simulink model "controller_3dof"  (R2023a)
settings: Solver=FixedStepAuto  StartTime=0.0  StopTime=inf  FixedStep=0.01  RelTol=1e-3  EnableMultiTasking=on
undefined symbols (not defined in the file): dev, DiscIntNeverNeededParam, IMU_w_b_bias, Kv, Kx, Main, meas_pole, P0_phth, P0_ps, pwm_output0, Q_phth, q_ps, R_phth, r_ps, Rz, Ts_EKF_integr, Ts_EKF_meas, Ts_slk, x0_phth, x0_ps
libraries: px4Sensorslib x4, px4lib x1, px4uORBlib x1, sharedtransform x1
settings Model: SimulationMode=external  ExtModeTrigDuration=10  Creator=ArriGE66  LastModifiedBy=User
settings SolverCC: PositivePriorityOrder=on
settings OptimizationCC: EnhancedBackFolding=on  PassReuseOutputArgsAs=Individual arguments  ZeroExternalMemoryAtStartup=off  ZeroInternalMemoryAtStartup=off  MaxStackSize=64  OptimizeBlockOrder=speed  DifferentSizesBufferReuse=on  OptimizationCustomize=off  EfficientTunableParamExpr=on
settings DebuggingCC: ParameterTunabilityLossMsg=error
settings HardwareCC: ProdBitPerPointer=32  ProdBitPerSizeT=32  ProdBitPerPtrDiffT=32  ProdLargestAtomicInteger=Long  ProdLargestAtomicFloat=Double  ProdWordSize=32  ProdLongLongMode=on  ProdHWDeviceType=ARM Compatible->ARM Cortex
settings SFSimCC: MATLABDynamicMemAlloc=off  SimTargetLang=C++
settings RTWCC: Description=Embedded Coder  SystemTargetFile=ert.tlc  HardwareBoard=PX4 Cube Orange  TemplateMakefile=ert_default_tmf  Toolchain=GNU Tools for PX4 Autopilots  TargetLang=C++
settings CodeAppCC: ForceParamTrailComments=on  IgnoreCustomStorageClasses=off  OperatorAnnotations=on  SimulinkDataObjDesc=on  SFDataObjDesc=on  InsertBlockDesc=on
settings ERTTargetCC: ExtMode=on  ExtModeTransport=3  ExtModeStaticAlloc=on  ExtModeStaticAllocSize=1024  ExtModeMexFile=ext_xcp  ExtModeMexArgs=1 COM10 3000000  ExtModeIntrfLevel=Level2 - Open

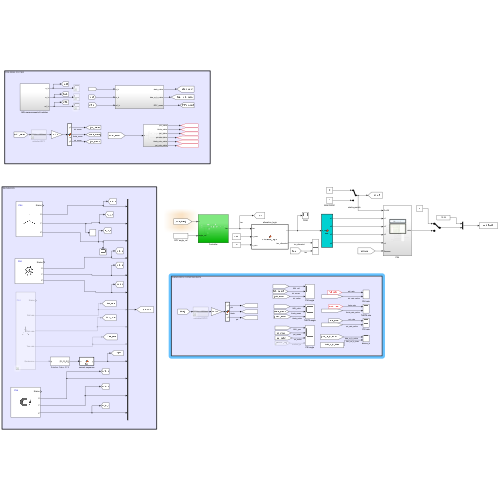
[thumbnail: Simulink's stored preview of the top-level diagram]
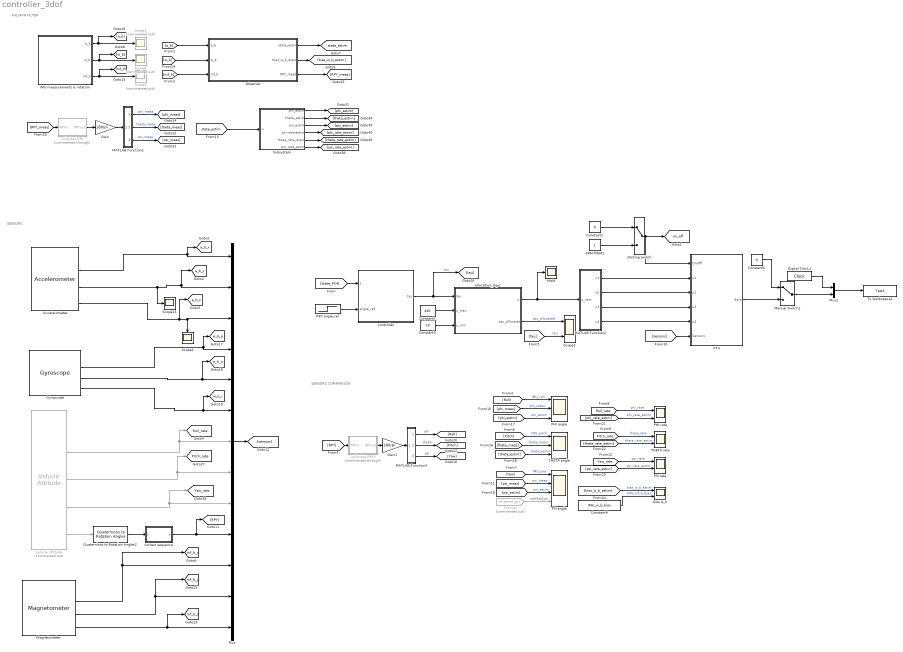
== system controller_3dof ==
  note: KALMAN FILTER
  note: SENSORS COMPARISON
  note: SENSORS
  ARM PWM1 : Constant  OutDataTypeStr=boolean  SampleTime=0.01
  Accelerometer : px4Sensorslib/Accelerometer  uorbTimeStamp=off  BlockingMode=off  BlockTimeout=1e-3  sampleTime=1/100
  Constant1 : Constant  Value=450  SampleTime=0.01
  Constant2 : Constant  Value=0  OutDataTypeStr=boolean
  Constant3 : Constant  Value=10  SampleTime=0.01
  Constant4 : Constant  Value=IMU_w_b_bias
  Constant6 : Constant  Value=0  OutDataTypeStr=boolean
  Controller : Subsystem
  Digital Clock1 : DigitalClock  SampleTime=0.01
  From20 : From  Commented=on  GotoTag=method_ps
  Gain : Gain  Gain=180/pi
  Gain1 : Gain  Gain=180/pi
  Gyroscope : px4Sensorslib/Gyroscope  uorbTimeStamp=off  BlockingMode=off  BlockTimeout=1e-3  sampleTime=1/100
  IMU measurements & rotation : Subsystem
  MATLAB Function1 : MATLAB Function  TreatAsAtomicUnit=on
  MATLAB Function2 : MATLAB Function  TreatAsAtomicUnit=on
  MATLAB Function3 : MATLAB Function  TreatAsAtomicUnit=on
  Magnetometer : px4Sensorslib/Magnetometer  uorbTimeStamp=off  BlockingMode=off  BlockTimeout=1e-3  sampleTime=0.01
  Manual Switch2 : ManualSwitch
  Mux : Mux  Inputs=13
  Mux2 : Mux  Inputs=2
  Observer : Subsystem
  PHI angle : Scope  NumInputPorts=3
  PHI rate : Scope  NumInputPorts=2
  PSI angle : Scope  NumInputPorts=4
  PSI rate : Scope  NumInputPorts=2
  PWM : Scope
  PX4 : Subsystem
  Quaternions to Rotation Angles2 : sharedtransform/Quaternions to Rotation Angles  rotationOrder=ZYX  aMode=aMode
  RPY angle_ref : Step  Time=0  After=zeros(3,1)  SampleTime=0.01
  Scope1 : Scope
  Scope13 : Scope
  Scope2 : Scope  NumInputPorts=2
  Scope3 : Scope  Commented=on
  Scope8 : Scope  Commented=on
  Scope9 : Scope  Commented=on
  Subsystem : Subsystem
  THETA angle : Scope  NumInputPorts=3
  THETA rate : Scope  NumInputPorts=2
  To Workspace1 : ToWorkspace  VariableName=Test1  SampleTime=-1
      settings: Save2DSignal=2-D array (concatenate along first dimension)
  Vehicle Attitude : px4Sensorslib/Vehicle Attitude  Commented=on  rollRate=on  pitchRate=on  yawRate=on  quaternion=on  uorbTimeStamp=off  BlockingMode=off  BlockTimeout=0.001  sampleTime=1/100
  allocation_logic : MATLAB Function  TreatAsAtomicUnit=on
  bias w_b : Scope  NumInputPorts=2
  correct sequence : MATLAB Function  TreatAsAtomicUnit=on
  starting switch : ManualSwitch
  unlimited RPY : Subsystem  Commented=through
  unlimited RPY2 : Subsystem  Commented=through
  tag scope: Pitch_rate=global, Roll_rate=global, Yaw_rate=global, a_b_x=global, a_b_y=global, a_b_z=global, mf_b_x=global, mf_b_y=global, mf_b_z=global, on_off=global, state_estim=global, w_b_p=global, w_b_q=global, w_b_r=global
  wires:
  MATLAB Function2/4(u4) -> PX4/5(u4)
  MATLAB Function2/3(u3) -> PX4/4(u3)
  MATLAB Function2/2(u2) -> PX4/3(u2)
  MATLAB Function2/1(u1) -> PX4/2(u1)
  allocation_logic/2(tau_allocated) -> Scope2/1  "tau_allocated"
  allocation_logic/1(u) -> PWM/1, MATLAB Function2/1(u_vect)
  Controller/1(tau) -> [tau], allocation_logic/1(tau)  "tau"
  RPY angle_ref/1 -> Controller/2(angle_ref)
  [tau] -> Scope2/2  "tau"
  [state_PX4] -> Controller/1(x)
  Constant3/1 -> allocation_logic/3(u_min)
  Subsystem/5(theta_rate_estim) -> [theta_rate_estim]
  Subsystem/6(psi_rate_estim) -> [psi_rate_estim]
  Subsystem/1(phi_estim) -> [phi_estim]
  Subsystem/3(psi_estim) -> [psi_estim]
  [state_estim] -> Subsystem/1(u)
  unlimited RPY2/1(RPYout) -> Gain1/1
  Observer/3(RPY_meas) -> [RPY_meas]
  IMU measurements & rotation/2(w_b) -> [w_b], Scope8/1
  MATLAB Function3/3(y3) -> [Yaw]  "psi"
  [theta_estim] -> THETA angle/3  "theta_estim"
  From20/1 -> PSI angle/4  "method_ps"
  [phi_rate_estim] -> PHI rate/2  "phi_rate_estim"
  Observer/1(state_estim) -> [state_estim]
  Mux/1 -> [sensors]
  starting switch/1 -> PX4/1(On/Off), [on_off]
  [Yaw] -> PSI angle/1  "IMU_yaw"
  Gyroscope/2 -> [w_b_p], Mux/4
  IMU measurements & rotation/3(mf_b) -> [mf_b], Scope9/1
  IMU measurements & rotation/1(a_b) -> [a_b], Scope3/1
  [w_b] -> Observer/2(w_b)
  [mf_b] -> Observer/3(mf_b)
  [a_b] -> Observer/1(a_b)
  [psi_rate_estim] -> PSI rate/2  "psi_rate_estim"
  unlimited RPY/1(RPYout) -> Gain/1
  Gyroscope/3 -> [w_b_q], Mux/5
  [Roll] -> PHI angle/1  "IMU_roll"
  [psi_estim] -> PSI angle/3  "psi_estim"
  [psi_meas] -> PSI angle/2  "psi_meas"
  Observer/2(bias_w_b_estim) -> [bias_w_b_estim]
  Constant4/1 -> bias w_b/2  "IMU_mf_b_bias"
  Manual Switch2/1 -> Mux2/2
  [phi_estim] -> PHI angle/3  "phi_estim"
  correct sequence/1(y) -> [RPY], Mux/10
  [RPY] -> unlimited RPY2/1(RPYin)
  Vehicle Attitude/5 -> Quaternions to Rotation Angles2/1
  [Pitch] -> THETA angle/1  "IMU_pitch"
  MATLAB Function3/2(y2) -> [Pitch]  "theta"
  Magnetometer/3 -> Mux/12, [mf_b_y]
  Gain1/1 -> MATLAB Function3/1(u)
  [Pitch_rate] -> THETA rate/1  "theta_rate"
  [bias_w_b_estim] -> bias w_b/1  "bias_w_b_estim"
  MATLAB Function1/1(y1) -> [phi_meas]  "phi_meas"
  [theta_rate_estim] -> THETA rate/2  "theta_rate_estim"
  [phi_meas] -> PHI angle/2  "phi_meas"
  Vehicle Attitude/2 -> [Roll_rate], Mux/7
  PX4/1(data) -> Manual Switch2/2
  Gain/1 -> MATLAB Function1/1(u)
  [RPY_meas] -> unlimited RPY/1(RPYin)
  Quaternions to Rotation Angles2/1 -> correct sequence/1(u)
  Subsystem/4(phi-rate-estim) -> [phi_rate_estim]
  Digital Clock1/1 -> Mux2/1
  Constant2/1 -> starting switch/1
  Vehicle Attitude/3 -> [Pitch_rate], Mux/8
  Constant6/1 -> Manual Switch2/1
  MATLAB Function1/3(y3) -> [psi_meas]  "psi_meas"
  [theta_meas] -> THETA angle/2  "theta_meas"
  Mux2/1 -> To Workspace1/1
  MATLAB Function1/2(y2) -> [theta_meas]  "theta_meas"
  [sensors] -> PX4/6(Sensors)
  Magnetometer/2 -> [mf_b_x], Mux/11
  Magnetometer/4 -> [mf_b_z], Mux/13
  [Yaw_rate] -> PSI rate/1  "psi_rate"
  Subsystem/2(theta_estim) -> [theta_estim]
  Vehicle Attitude/4 -> [Yaw_rate], Mux/9
  Gyroscope/4 -> [w_b_r], Mux/6
  Accelerometer/3 -> Scope13/1, [a_b_y], Mux/2
  MATLAB Function3/1(y1) -> [Roll]  "phi"
  ARM PWM1/1 -> starting switch/2
  [Roll_rate] -> PHI rate/1  "phi_rate"
  Accelerometer/2 -> [a_b_x], Mux/1
  Accelerometer/4 -> [a_b_z], Mux/3, Scope1/1
  Constant1/1 -> allocation_logic/2(u_max)

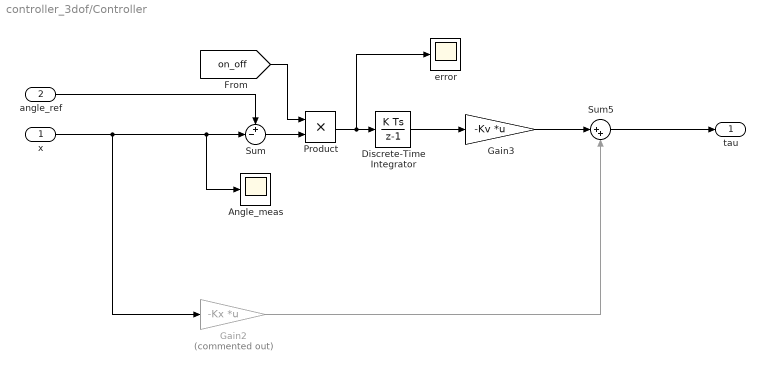
== system controller_3dof/Controller ==
  x : Inport
  angle_ref : Inport  Port=2
  Angle_meas : Scope
  Discrete-Time Integrator : DiscreteIntegrator  SampleTime=Ts_slk  ICPrevOutput=DiscIntNeverNeededParam  ICPrevScaledInput=DiscIntNeverNeededParam
  Gain2 : Gain  Commented=on  Gain=-Kx  Multiplication=Matrix(K*u)
  Gain3 : Gain  Gain=-Kv  Multiplication=Matrix(K*u)
  Product : Product
  Sum : Sum  Inputs=+-|
  Sum5 : Sum  Inputs=|++
  error : Scope
  tau : Outport
  wires:
  x/1 -> Angle_meas/1, Sum/2, Gain2/1
  Sum5/1 -> tau/1
  angle_ref/1 -> Sum/1
  Discrete-Time Integrator/1 -> Gain3/1
  Gain3/1 -> Sum5/1
  Gain2/1 -> Sum5/2
  Sum/1 -> Product/2
  [on_off] -> Product/1
  Product/1 -> error/1, Discrete-Time Integrator/1

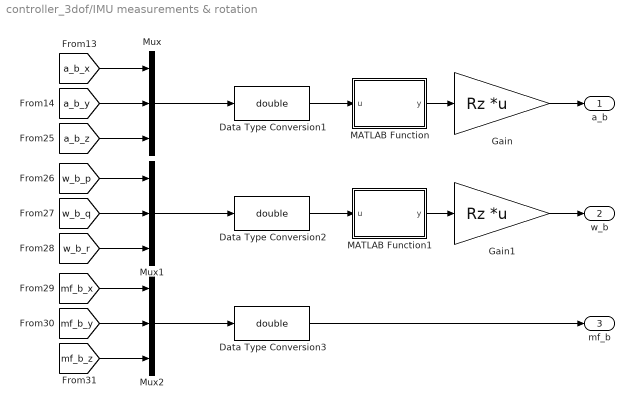
== system controller_3dof/IMU measurements & rotation ==
  Data Type Conversion1 : DataTypeConversion  OutDataTypeStr=double  SaturateOnIntegerOverflow=off  RndMeth=Floor
  Data Type Conversion2 : DataTypeConversion  OutDataTypeStr=double  SaturateOnIntegerOverflow=off  RndMeth=Floor
  Data Type Conversion3 : DataTypeConversion  OutDataTypeStr=double  SaturateOnIntegerOverflow=off  RndMeth=Floor
  Gain : Gain  Gain=Rz  Multiplication=Matrix(K*u) (u vector)
  Gain1 : Gain  Gain=Rz  Multiplication=Matrix(K*u) (u vector)
  MATLAB Function : MATLAB Function  TreatAsAtomicUnit=on
  MATLAB Function1 : MATLAB Function  TreatAsAtomicUnit=on
  Mux : Mux  Inputs=3
  Mux1 : Mux  Inputs=3
  Mux2 : Mux  Inputs=3
  a_b : Outport
  w_b : Outport  Port=2
  mf_b : Outport  Port=3
  wires:
  Mux2/1 -> Data Type Conversion3/1
  Gain/1 -> a_b/1
  Mux1/1 -> Data Type Conversion2/1
  MATLAB Function/1(y) -> Gain/1
  Mux/1 -> Data Type Conversion1/1
  MATLAB Function1/1(y) -> Gain1/1
  Gain1/1 -> w_b/1
  [a_b_x] -> Mux/1
  [a_b_y] -> Mux/2
  [a_b_z] -> Mux/3
  [w_b_p] -> Mux1/1
  [w_b_q] -> Mux1/2
  [w_b_r] -> Mux1/3
  [mf_b_x] -> Mux2/1
  [mf_b_y] -> Mux2/2
  [mf_b_z] -> Mux2/3
  Data Type Conversion1/1 -> MATLAB Function/1(u)
  Data Type Conversion2/1 -> MATLAB Function1/1(u)
  Data Type Conversion3/1 -> mf_b/1

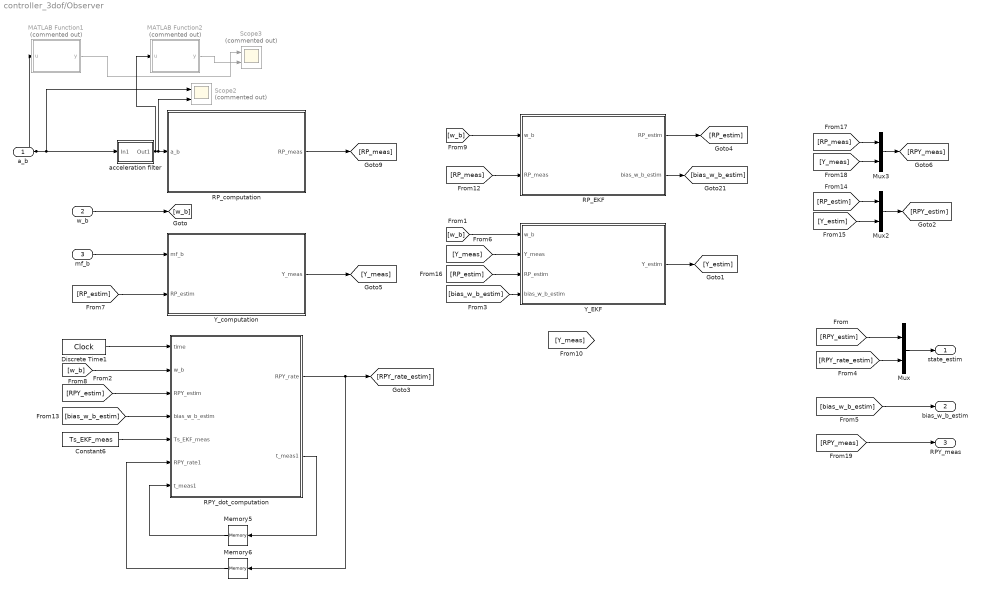
== system controller_3dof/Observer ==
  a_b : Inport
  w_b : Inport  Port=2
  mf_b : Inport  Port=3
  Constant6 : Constant  Value=Ts_EKF_meas
  Discrete Time1 : DigitalClock  SampleTime=Ts_slk
  MATLAB Function1 : MATLAB Function  Commented=on  TreatAsAtomicUnit=on
  MATLAB Function2 : MATLAB Function  Commented=on  TreatAsAtomicUnit=on
  Memory5 : Memory
  Memory6 : Memory
  Mux : Mux  Inputs=2
  Mux2 : Mux  Inputs=2
  Mux3 : Mux  Inputs=2
  RPY_dot_computation : MATLAB Function  TreatAsAtomicUnit=on
  RP_EKF : Subsystem
  RP_computation : MATLAB Function  TreatAsAtomicUnit=on
  Scope2 : Scope  Commented=on  NumInputPorts=2
  Scope3 : Scope  Commented=on  NumInputPorts=2
  Y_EKF : Subsystem
  Y_computation : MATLAB Function  TreatAsAtomicUnit=on
  acceleration filter : Subsystem  mask{p=meas_pole}
      mask prompts: p "pole (p)"
  state_estim : Outport
  bias_w_b_estim : Outport  Port=2
  RPY_meas : Outport  Port=3
  wires:
  Memory5/1 -> RPY_dot_computation/7("t_meas1 ")
  Discrete Time1/1 -> RPY_dot_computation/1(time)
  RPY_dot_computation/2(t_meas1) -> Memory5/1
  [w_b] -> RPY_dot_computation/2(w_b)
  Memory6/1 -> RPY_dot_computation/6(RPY_rate1)
  RPY_dot_computation/1(RPY_rate) -> Memory6/1, [RPY_rate_estim]
  Constant6/1 -> RPY_dot_computation/5(Ts_EKF_meas)
  [RPY_estim] -> RPY_dot_computation/3(RPY_estim)
  [bias_w_b_estim] -> RPY_dot_computation/4(bias_w_b_estim)
  [RPY_estim] -> Mux/1
  [RPY_rate_estim] -> Mux/2
  Mux/1 -> state_estim/1
  [bias_w_b_estim] -> bias_w_b_estim/1
  [RPY_meas] -> RPY_meas/1
  RP_EKF/2(bias_w_b_estim) -> [bias_w_b_estim]
  [RP_estim] -> Y_computation/2(RP_estim)
  [Y_meas] -> Y_EKF/2(Y_meas)
  Y_computation/1(Y_meas) -> [Y_meas]
  RP_EKF/1(RP_estim) -> [RP_estim]
  [w_b] -> Y_EKF/1(w_b)
  RP_computation/1(RP_meas) -> [RP_meas]
  [RP_meas] -> RP_EKF/2(RP_meas)
  [w_b] -> RP_EKF/1(w_b)
  Y_EKF/1(Y_estim) -> [Y_estim]
  mf_b/1 -> Y_computation/1(mf_b)
  w_b/1 -> [w_b]
  [bias_w_b_estim] -> Y_EKF/4(bias_w_b_estim)
  [RP_estim] -> Mux2/1
  [Y_estim] -> Mux2/2
  Mux2/1 -> [RPY_estim]
  [RP_estim] -> Y_EKF/3(RP_estim)
  [RP_meas] -> Mux3/1
  Mux3/1 -> [RPY_meas]
  [Y_meas] -> Mux3/2
  MATLAB Function1/1(y) -> Scope3/1
  a_b/1 -> Scope2/1, acceleration filter/1(In1), MATLAB Function1/1(u)
  MATLAB Function2/1(y) -> Scope3/2
  acceleration filter/1(Out1) -> MATLAB Function2/1(u), Scope2/2, RP_computation/1(a_b)

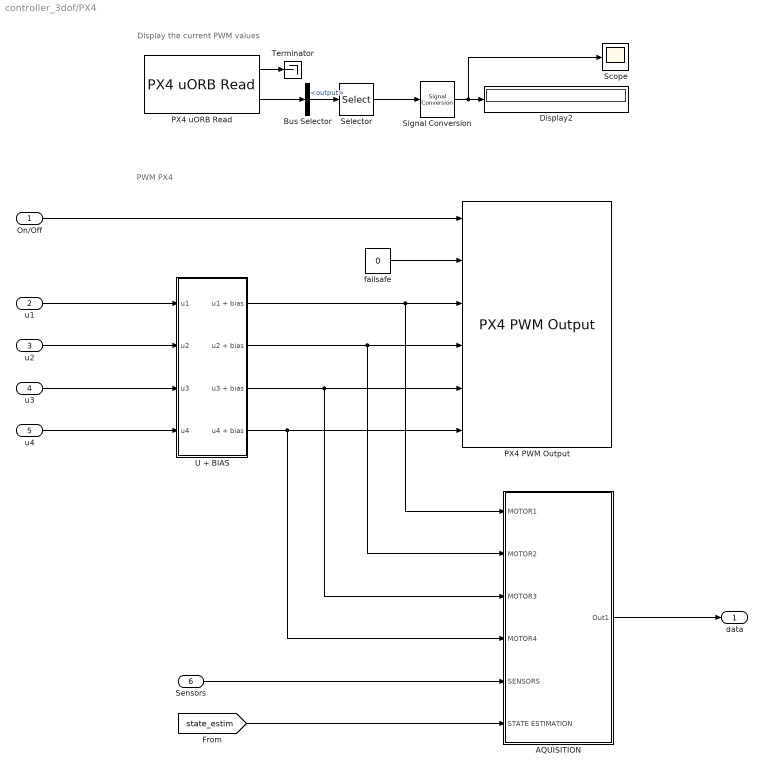
== system controller_3dof/PX4 ==
  note: PWM PX4
  note: Display the current PWM values
  On/Off : Inport
  u1 : Inport  Port=2
  u2 : Inport  Port=3
  u3 : Inport  Port=4
  u4 : Inport  Port=5
  Sensors : Inport  Port=6
  AQUISITION : Subsystem
  Bus Selector : BusSelector  OutputSignals=output
  Display2 : Display
  PX4 PWM Output : px4lib/PX4 PWM Output  pwmDevice=Main (/dev/pwm_output0)  pwmChannel1_=on  pwmChannel2_=on  pwmChannel3_=on  pwmChannel4_=on  pwmChannel5_=off  pwmChannel6_=off  pwmChannel7_=off  pwmChannel8_=off  forceTerminateFailsafe=off  outputErrorStatus=on
  PX4 uORB Read : px4uORBlib/PX4 uORB Read  uORBTopic=actuator_outputs  selectInstance=actuator_outputs  SampleTime=0.01  BlockingMode=off  BlockTimeout=1e-3
  Scope : Scope
  Selector : Selector  InputPortWidth=16  IndexOptions=Index vector (dialog)  Indices=[1 2]  OutputSizes=1
  Signal Conversion : SignalConversion  OverrideOpt=off
  Terminator : Terminator
  U + BIAS : Subsystem
  failsafe : Constant  Value=0  OutDataTypeStr=boolean  SampleTime=0.01
  data : Outport
  wires:
  failsafe/1 -> PX4 PWM Output/2
  U + BIAS/2(u2 + bias) -> AQUISITION/2(MOTOR2), PX4 PWM Output/4
  U + BIAS/4(u4 + bias) -> AQUISITION/4(MOTOR4), PX4 PWM Output/6
  U + BIAS/3(u3 + bias) -> AQUISITION/3(MOTOR3), PX4 PWM Output/5
  U + BIAS/1(u1 + bias) -> AQUISITION/1(MOTOR1), PX4 PWM Output/3
  Sensors/1 -> AQUISITION/5(SENSORS)
  On/Off/1 -> PX4 PWM Output/1
  u4/1 -> U + BIAS/4(u4)
  AQUISITION/1(Out1) -> data/1
  u1/1 -> U + BIAS/1(u1)
  u2/1 -> U + BIAS/2(u2)
  u3/1 -> U + BIAS/3(u3)
  [state_estim] -> AQUISITION/6(STATE ESTIMATION)
  Selector/1 -> Signal Conversion/1
  PX4 uORB Read/2 -> Bus Selector/1
  Signal Conversion/1 -> Scope/1, Display2/1
  Bus Selector/1 -> Selector/1  "<output>"
  PX4 uORB Read/1 -> Terminator/1

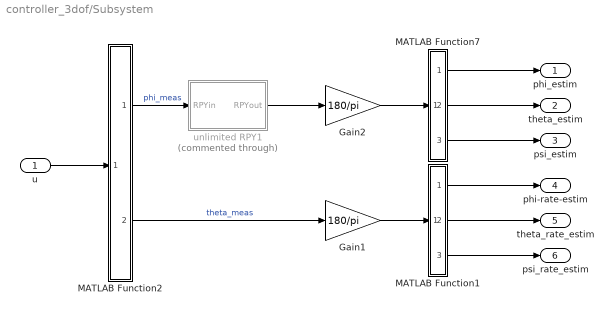
== system controller_3dof/Subsystem ==
  u : Inport
  Gain1 : Gain  Gain=180/pi
  Gain2 : Gain  Gain=180/pi
  MATLAB Function1 : MATLAB Function  TreatAsAtomicUnit=on
  MATLAB Function2 : MATLAB Function  TreatAsAtomicUnit=on
  MATLAB Function7 : MATLAB Function  TreatAsAtomicUnit=on
  unlimited RPY1 : Subsystem  Commented=through
  phi_estim : Outport
  theta_estim : Outport  Port=2
  psi_estim : Outport  Port=3
  phi-rate-estim : Outport  Port=4
  theta_rate_estim : Outport  Port=5
  psi_rate_estim : Outport  Port=6
  wires:
  u/1 -> MATLAB Function2/1(u)
  MATLAB Function2/2(y2) -> Gain1/1  "theta_meas"
  MATLAB Function2/1(y1) -> unlimited RPY1/1(RPYin)  "phi_meas"
  MATLAB Function7/2(y2) -> theta_estim/1
  MATLAB Function7/1(y1) -> phi_estim/1
  MATLAB Function7/3(y3) -> psi_estim/1
  unlimited RPY1/1(RPYout) -> Gain2/1
  Gain2/1 -> MATLAB Function7/1(u)
  Gain1/1 -> MATLAB Function1/1(u)
  MATLAB Function1/3(y3) -> psi_rate_estim/1
  MATLAB Function1/2(y2) -> theta_rate_estim/1
  MATLAB Function1/1(y1) -> phi-rate-estim/1

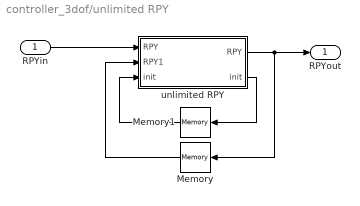
== system controller_3dof/unlimited RPY ==
  RPYin : Inport
  Memory : Memory
  Memory1 : Memory
  unlimited RPY : MATLAB Function  TreatAsAtomicUnit=on
  RPYout : Outport
  wires:
  RPYin/1 -> unlimited RPY/1("RPY ")
  unlimited RPY/1(RPY) -> Memory/1, RPYout/1
  Memory/1 -> unlimited RPY/2(RPY1)
  unlimited RPY/2(init) -> Memory1/1
  Memory1/1 -> unlimited RPY/3("init ")

== system controller_3dof/unlimited RPY2 ==
  RPYin : Inport
  Memory : Memory
  Memory1 : Memory
  unlimited RPY : MATLAB Function  TreatAsAtomicUnit=on
  RPYout : Outport
  wires:
  RPYin/1 -> unlimited RPY/1("RPY ")
  unlimited RPY/1(RPY) -> Memory/1, RPYout/1
  Memory/1 -> unlimited RPY/2(RPY1)
  unlimited RPY/2(init) -> Memory1/1
  Memory1/1 -> unlimited RPY/3("init ")

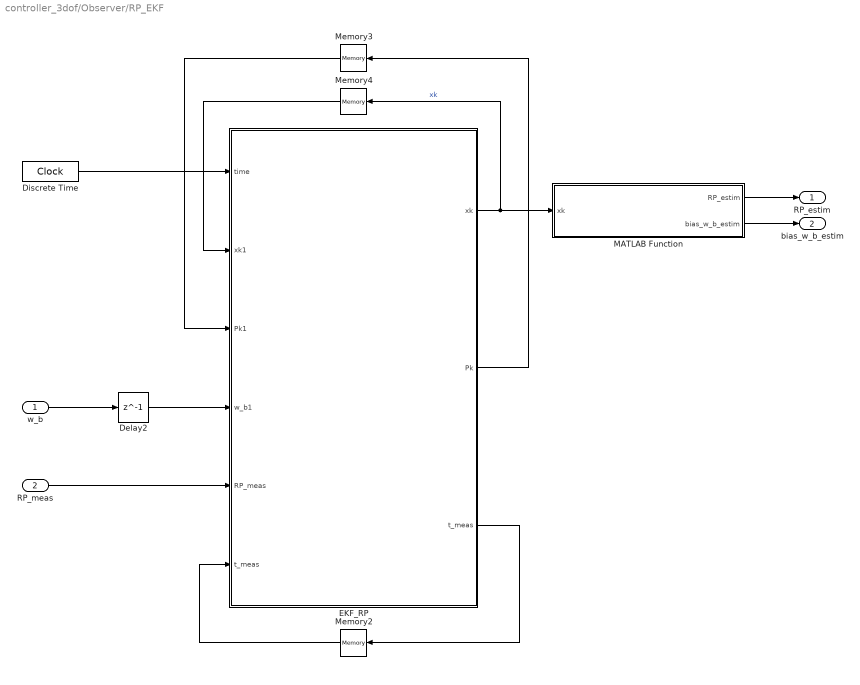
== system controller_3dof/Observer/RP_EKF ==
  w_b : Inport
  RP_meas : Inport  Port=2
  Delay2 : Delay  DelayLength=1  SampleTime=Ts_EKF_meas
  Discrete Time : DigitalClock  SampleTime=Ts_slk
  EKF_RP : MATLAB Function  TreatAsAtomicUnit=on
  MATLAB Function : MATLAB Function  TreatAsAtomicUnit=on
  Memory2 : Memory
  Memory3 : Memory  InitialCondition=P0_phth
  Memory4 : Memory  InitialCondition=x0_phth
  RP_estim : Outport
  bias_w_b_estim : Outport  Port=2
  wires:
  w_b/1 -> Delay2/1
  EKF_RP/2(Pk) -> Memory3/1
  Memory2/1 -> EKF_RP/6("t_meas ")
  EKF_RP/3(t_meas) -> Memory2/1
  RP_meas/1 -> EKF_RP/5(RP_meas)
  Discrete Time/1 -> EKF_RP/1(time)
  Memory3/1 -> EKF_RP/3(Pk1)
  Delay2/1 -> EKF_RP/4(w_b1)
  Memory4/1 -> EKF_RP/2(xk1)
  EKF_RP/1(xk) -> Memory4/1, MATLAB Function/1(xk)  "xk"
  MATLAB Function/1(RP_estim) -> RP_estim/1
  MATLAB Function/2(bias_w_b_estim) -> bias_w_b_estim/1

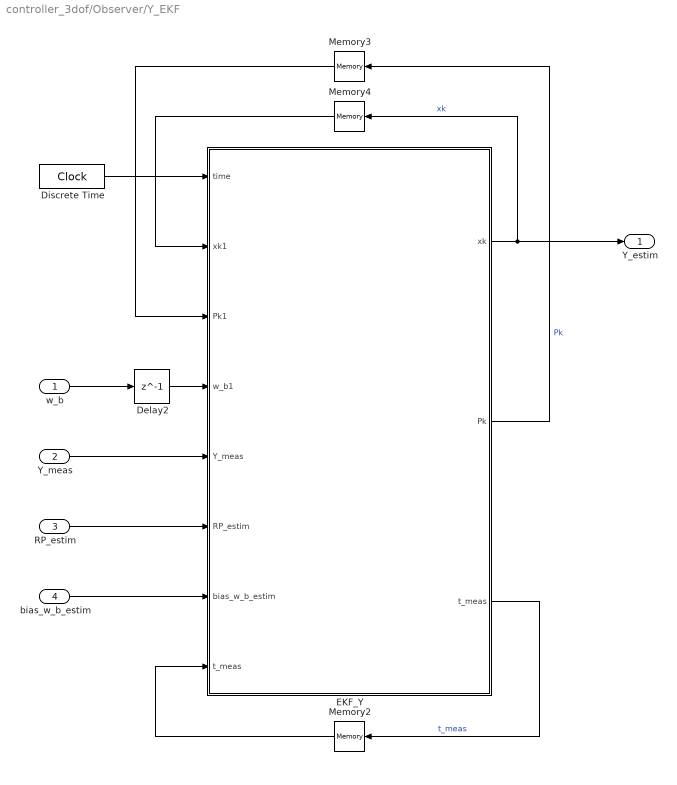
== system controller_3dof/Observer/Y_EKF ==
  w_b : Inport
  Y_meas : Inport  Port=2
  RP_estim : Inport  Port=3
  bias_w_b_estim : Inport  Port=4
  Delay2 : Delay  DelayLength=1  SampleTime=Ts_EKF_meas
  Discrete Time : DigitalClock  SampleTime=Ts_slk
  EKF_Y : MATLAB Function  TreatAsAtomicUnit=on
  Memory2 : Memory
  Memory3 : Memory  InitialCondition=ones(1,1)*P0_ps
  Memory4 : Memory  InitialCondition=ones(1,1)*x0_ps
  Y_estim : Outport
  wires:
  w_b/1 -> Delay2/1
  EKF_Y/2(Pk) -> Memory3/1  "Pk"
  Memory2/1 -> EKF_Y/8("t_meas ")
  EKF_Y/3(t_meas) -> Memory2/1  "t_meas"
  Y_meas/1 -> EKF_Y/5(Y_meas)
  Discrete Time/1 -> EKF_Y/1(time)
  Memory3/1 -> EKF_Y/3(Pk1)
  Delay2/1 -> EKF_Y/4(w_b1)
  Memory4/1 -> EKF_Y/2(xk1)
  EKF_Y/1(xk) -> Memory4/1, Y_estim/1  "xk"
  bias_w_b_estim/1 -> EKF_Y/7(bias_w_b_estim)
  RP_estim/1 -> EKF_Y/6(RP_estim)

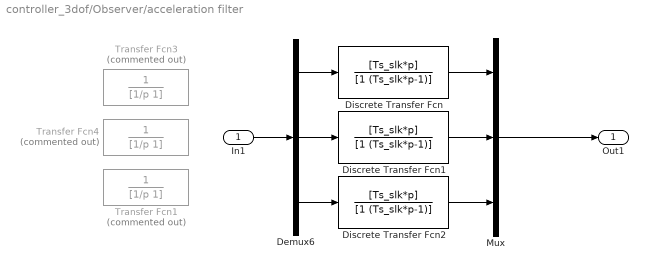
== system controller_3dof/Observer/acceleration filter ==
  In1 : Inport
  Demux6 : Demux  Outputs=3
  Discrete Transfer Fcn : DiscreteTransferFcn  Numerator=[Ts_slk*p]  Denominator=[1 (Ts_slk*p-1)]
  Discrete Transfer Fcn1 : DiscreteTransferFcn  Numerator=[Ts_slk*p]  Denominator=[1 (Ts_slk*p-1)]
  Discrete Transfer Fcn2 : DiscreteTransferFcn  Numerator=[Ts_slk*p]  Denominator=[1 (Ts_slk*p-1)]
  Mux : Mux  Inputs=3
  Transfer Fcn1 : TransferFcn  Commented=on  Denominator=[1/p 1]
  Transfer Fcn3 : TransferFcn  Commented=on  Denominator=[1/p 1]
  Transfer Fcn4 : TransferFcn  Commented=on  Denominator=[1/p 1]
  Out1 : Outport
  wires:
  Discrete Transfer Fcn1/1 -> Mux/2
  Demux6/3 -> Discrete Transfer Fcn2/1
  Mux/1 -> Out1/1
  Discrete Transfer Fcn2/1 -> Mux/3
  Discrete Transfer Fcn/1 -> Mux/1
  In1/1 -> Demux6/1
  Demux6/1 -> Discrete Transfer Fcn/1
  Demux6/2 -> Discrete Transfer Fcn1/1

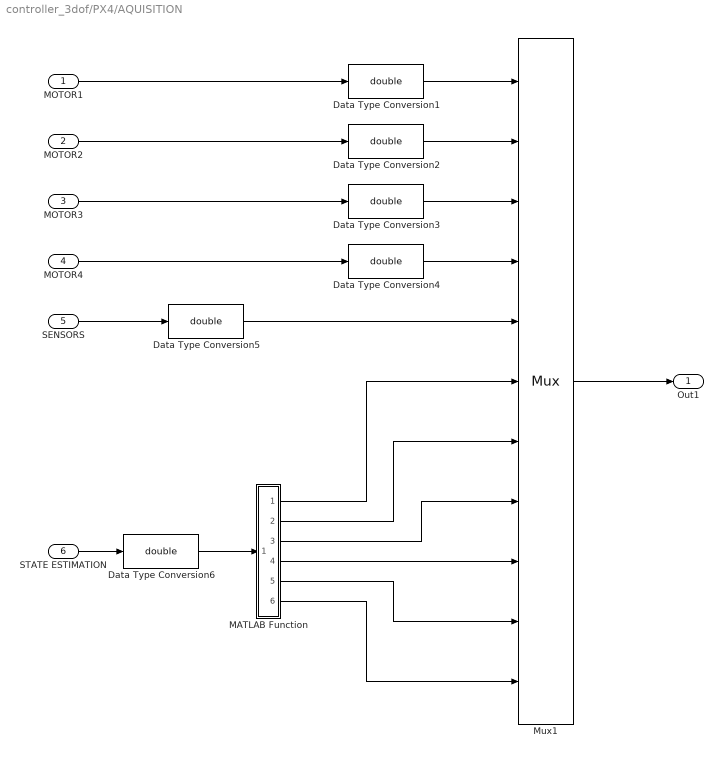
== system controller_3dof/PX4/AQUISITION ==
  MOTOR1 : Inport
  MOTOR2 : Inport  Port=2
  MOTOR3 : Inport  Port=3
  MOTOR4 : Inport  Port=4
  SENSORS : Inport  Port=5
  STATE ESTIMATION : Inport  Port=6
  Data Type Conversion{1..6} (6 alike) : DataTypeConversion  OutDataTypeStr=double  SaturateOnIntegerOverflow=off  RndMeth=Floor
  MATLAB Function : MATLAB Function  TreatAsAtomicUnit=on
  Mux1 : Mux  Inputs=11
      settings: DisplayOption=signals
  Out1 : Outport
  wires:
  MOTOR2/1 -> Data Type Conversion2/1
  Data Type Conversion1/1 -> Mux1/1
  Data Type Conversion3/1 -> Mux1/3
  Data Type Conversion4/1 -> Mux1/4
  Data Type Conversion2/1 -> Mux1/2
  MOTOR3/1 -> Data Type Conversion3/1
  STATE ESTIMATION/1 -> Data Type Conversion6/1
  Mux1/1 -> Out1/1
  SENSORS/1 -> Data Type Conversion5/1
  MOTOR1/1 -> Data Type Conversion1/1
  MOTOR4/1 -> Data Type Conversion4/1
  MATLAB Function/1(y1) -> Mux1/6
  MATLAB Function/6(y6) -> Mux1/11
  MATLAB Function/5(y5) -> Mux1/10
  MATLAB Function/4(y4) -> Mux1/9
  MATLAB Function/2(y2) -> Mux1/7
  Data Type Conversion6/1 -> MATLAB Function/1(u)
  MATLAB Function/3(y3) -> Mux1/8
  Data Type Conversion5/1 -> Mux1/5

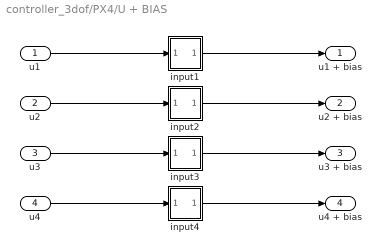
== system controller_3dof/PX4/U + BIAS ==
  u1 : Inport
  u2 : Inport  Port=2
  u3 : Inport  Port=3
  u4 : Inport  Port=4
  input1 : Subsystem
  input2 : Subsystem
  input3 : Subsystem
  input4 : Subsystem
  u1 + bias : Outport
  u2 + bias : Outport  Port=2
  u3 + bias : Outport  Port=3
  u4 + bias : Outport  Port=4
  wires:
  u2/1 -> input2/1(In1)
  u1/1 -> input1/1(In1)
  input1/1(Out1) -> u1 + bias/1
  u4/1 -> input4/1(In1)
  input4/1(Out1) -> u4 + bias/1
  input2/1(Out1) -> u2 + bias/1
  u3/1 -> input3/1(In1)
  input3/1(Out1) -> u3 + bias/1

== system controller_3dof/Subsystem/unlimited RPY1 ==
  RPYin : Inport
  Memory : Memory
  Memory1 : Memory
  unlimited RPY : MATLAB Function  TreatAsAtomicUnit=on
  RPYout : Outport
  wires:
  RPYin/1 -> unlimited RPY/1("RPY ")
  unlimited RPY/1(RPY) -> Memory/1, RPYout/1
  Memory/1 -> unlimited RPY/2(RPY1)
  unlimited RPY/2(init) -> Memory1/1
  Memory1/1 -> unlimited RPY/3("init ")

== system controller_3dof/PX4/U + BIAS/input1 ==
  In1 : Inport
  Constant : Constant  Value=1000  SampleTime=0.01
  Data Type Conversion1 : DataTypeConversion  OutDataTypeStr=uint16  SaturateOnIntegerOverflow=off  RndMeth=Floor
  Sum : Sum  Inputs=|++
  Out1 : Outport
  wires:
  Sum/1 -> Data Type Conversion1/1
  In1/1 -> Sum/1
  Constant/1 -> Sum/2
  Data Type Conversion1/1 -> Out1/1

== system controller_3dof/PX4/U + BIAS/input2 ==
  In1 : Inport
  Constant : Constant  Value=1000  SampleTime=0.01
  Data Type Conversion1 : DataTypeConversion  OutDataTypeStr=uint16  SaturateOnIntegerOverflow=off  RndMeth=Floor
  Sum : Sum  Inputs=|++
  Out1 : Outport
  wires:
  Sum/1 -> Data Type Conversion1/1
  In1/1 -> Sum/1
  Constant/1 -> Sum/2
  Data Type Conversion1/1 -> Out1/1

== system controller_3dof/PX4/U + BIAS/input3 ==
  In1 : Inport
  Constant : Constant  Value=1200  SampleTime=0.01
  Data Type Conversion1 : DataTypeConversion  OutDataTypeStr=uint16  SaturateOnIntegerOverflow=off  RndMeth=Floor
  Sum : Sum  Inputs=|++
  Out1 : Outport
  wires:
  Sum/1 -> Data Type Conversion1/1
  In1/1 -> Sum/1
  Constant/1 -> Sum/2
  Data Type Conversion1/1 -> Out1/1

== system controller_3dof/PX4/U + BIAS/input4 ==
  In1 : Inport
  Constant : Constant  Value=1000  SampleTime=0.01
  Data Type Conversion1 : DataTypeConversion  OutDataTypeStr=uint16  SaturateOnIntegerOverflow=off  RndMeth=Floor
  Sum : Sum  Inputs=|++
  Out1 : Outport
  wires:
  Sum/1 -> Data Type Conversion1/1
  In1/1 -> Sum/1
  Constant/1 -> Sum/2
  Data Type Conversion1/1 -> Out1/1

== matlab function controller_3dof/Subsystem/MATLAB Function2 ==
  data: u input; y1 output; y2 output
function [y1,y2] = fcn(u)

y1 = u(1:3);
y2 = u(4:6);
end

== matlab function controller_3dof/correct sequence ==
  data: u input; y output
function y  = fcn(u)

y = single([0,0,0]);
y(1) = u(3);
y(2) = u(2);
y(3) = u(1);

== matlab function controller_3dof/Observer/RPY_dot_computation ==
  data: time input; w_b input; RPY_estim input; bias_w_b_estim input; Ts_EKF_meas input; RPY_rate1 input; RPY_rate output; t_meas1 input; t_meas1 output
function [RPY_rate,t_meas1] = RPY_dot_computation(time,w_b,RPY_estim,bias_w_b_estim,Ts_EKF_meas,RPY_rate1,t_meas1)

if time - t_meas1 >= Ts_EKF_meas || time == 0
    wp          =       w_b(1,1);               % p-dir of angular velocity w
    wq          =       w_b(2,1);               % q-dir of angular velocity w
    wr          =       w_b(3,1);               % r-dir of angular velocity w

    phi         =       RPY_estim(1,1);         % roll angle (rad)
    theta       =       RPY_estim(2,1);         % pitch angle (rad)
    psi         =       RPY_estim(3,1);         % yaw angle (rad)  
    bias_wp     =       bias_w_b_estim(1,1)*0;    % bias of p-dir of angular velocity w
    bias_wq     =       bias_w_b_estim(2,1)*0;    % bias of q-dir of angular velocity w
    bias_wr     =       bias_w_b_estim(3,1)*0;   % bias of r-dir of angular velocity w

    cph         =       cos(phi);
    cth         =       cos(theta);
    cps         =       cos(psi);
    sph         =       sin(phi);
    sth         =       sin(theta);
    sps         =       sin(psi);
    tth         =       sth/cth;

    % integration step
    t_meas1 = time;
    W_eta = [1,    sph*tth,    cph*tth;
             0,    cph,        -sph;
             0,    sph/cth,    cph/cth;];
    w_b_corrected = [wp-bias_wp; wq-bias_wq; wr-bias_wr;];
    RPY_rate = W_eta*w_b_corrected;
else
    RPY_rate = RPY_rate1;
end
end

== matlab function controller_3dof/Observer/RP_EKF/EKF_RP ==
  data: time input; xk1 input; Pk1 input; w_b1 input; RP_meas input; t_meas input; Q_phth parameter; xk output; Pk output; t_meas output; R_phth parameter; Ts_EKF_integr parameter; Ts_EKF_meas parameter
function [xk,Pk,t_meas] = EKF_RP(time,xk1,Pk1,w_b1,RP_meas,t_meas,Q_phth,R_phth,Ts_EKF_integr,Ts_EKF_meas)

if time - t_meas >= Ts_EKF_meas
    t_meas = time;
    Q = Q_phth;
    R = R_phth;

  % INTEGRATION STEP
    % initial condition
    xt1         =       xk1;                        % initial condition for the state
    Pt1         =       Pk1;                        % initial condition for matrix P
    wp1         =       w_b1(1,1);                  % past value of the p-dir of angular velocity w
    wq1         =       w_b1(2,1);                  % past value of the q-dir of angular velocity w
    wr1         =       w_b1(3,1);                  % past value of the r-dir of angular velocity w
    % integration loop
    Nstep       = floor(Ts_EKF_meas/Ts_EKF_integr); % number of integration steps to performe in the t_meas time windows
    xt          = zeros(5,1);
    Pt          = zeros(5,5);
    for i = 1:1:Nstep
        % state extraction
            phi         =       xt1(1,1);           % roll angle (rad)
            theta       =       xt1(2,1);           % pitch angle (rad)  
            bias_wp     =       xt1(3,1);           % bias of p-dir of angular velocity w
            bias_wq     =       xt1(4,1);           % bias of q-dir of angular velocity w
            bias_wr     =       xt1(5,1);           % bias of r-dir of angular velocity w
        
            cph         =       cos(phi);
            cth         =       cos(theta);
            sph         =       sin(phi);
            sth         =       sin(theta);
            tth         =       sth/cth;
        % integration
            Mf = [1,    sph*tth,    cph*tth,    0,  0,  0;
                  0,    cph,        -sph,       0,  0,  0;
                  0,    0,          0,          0,  0,  0;
                  0,    0,          0,          0,  0,  0;
                  0,    0,          0,          0,  0,  0;];
            Z1 = [wp1-bias_wp; wq1-bias_wq; wr1-bias_wr; bias_wp; bias_wq; bias_wr;];
            f = Mf*Z1;
            xt = xt1 + Ts_EKF_integr*f;
        
            A1 = [cph*tth*(wq1-bias_wq)-sph*tth*(wr1-bias_wr),(sph*(wq1-bias_wq)+cph*(wr1-bias_wr))/cth^2,  -1, -sph*tth,   -cph*tth;];
            A2 = [-sph*(wq1-bias_wq)-cph*(wr1-bias_wr),  0,  0,  -cph,   sph;];
            A3 = [0,  0,  0,  0,  0;];
            A4 = [0,  0,  0,  0,  0;];
            A5 = [0,  0,  0,  0,  0;];
            At1 = [A1; A2; A3; A4; A5;];
            Pt = Pt1 + Ts_EKF_integr*(At1*Pt1 + Pt1*At1' + Q);
        % house keeping
            xt1 = xt;
            Pt1 = Pt;
    end
  % MEASUREMENT STEP
    Ck = [eye(2),zeros(2,3)];
    Lk = Pt*Ck'/(Ck*Pt*Ck' + R);
    xk = xt + Lk*(RP_meas - Ck*xt);
    Pk = (eye(5) - Lk*Ck)*Pt;
else
    xk = xk1;
    Pk = Pk1;
end
end

== matlab function controller_3dof/Observer/RP_EKF/MATLAB Function ==
  data: xk input; RP_estim output; bias_w_b_estim output
function [RP_estim, bias_w_b_estim] = state_extraction(xk)

RP_estim        = xk(1:2,1);
bias_w_b_estim  = xk(3:5,1);
end

== matlab function controller_3dof/Observer/RP_computation ==
  data: a_b input; RP_meas output
function RP_meas    = RP_computation(a_b)
% description:
% - a_b             = measured linear acceleration in body-frame
% - w_b             = measured angular velocity in body-frame
% - mf_b            = measured magnetic field in body-frame
% - mf              = measured magnetic field in body-inertia
% - a_b_disturbe    = linear velocity measurement-noise
% - w_b_disturbe    = angular velocity measurement-noise
% - mf_b_disturbe   = magnetic field measurement-noise

% -------------------------------------------------------------------------------------------
% observation: the following computation works only if the angles
% phi,theta,psy are withing angles (-pi/2,+pi/2) (this is an open set, pi/2 is excluded)
% -------------------------------------------------------------------------------------------

a_b = -1*a_b;       % need to adjust the sign to use atan2() function correctly

% phi computation
ph_meas = atan2(a_b(2), a_b(3));
sph = sin(ph_meas);
cph = cos(ph_meas);

% theta computation
th_meas = atan2(-a_b(1), (a_b(2)*sph + a_b(3)*cph));

RP_meas = [ph_meas;th_meas];

== matlab function controller_3dof/Observer/Y_EKF/EKF_Y ==
  data: time input; xk1 input size=[1,1]; Pk1 input size=[1,1]; w_b1 input; Y_meas input; RP_estim input; bias_w_b_estim input; t_meas input; q_ps parameter; xk output size=[1,1]; Pk output; t_meas output; r_ps parameter; Ts_EKF_integr parameter; Ts_EKF_meas parameter
function [xk,Pk,t_meas] = EKF_Y(time,xk1,Pk1,w_b1,Y_meas,RP_estim,bias_w_b_estim,t_meas,q_ps,r_ps,Ts_EKF_integr,Ts_EKF_meas)

if time - t_meas >= Ts_EKF_meas
    t_meas = time;
    Q = q_ps;
    R = r_ps;

  % INTEGRATION STEP
    % initial condition
    xt1         =       xk1;                        % initial condition for the state
    Pt1         =       Pk1;                        % initial condition for matrix P

    wp1         =       w_b1(1,1);                  % past value of the p-dir of angular velocity w
    wq1         =       w_b1(2,1);                  % past value of the q-dir of angular velocity w
    wr1         =       w_b1(3,1);                  % past value of the r-dir of angular velocity w

    phi         =       RP_estim(1,1);              % estimate of roll angle (rad)
    theta       =       RP_estim(2,1);              % estimate of pitch angle (rad)  

    bias_wp     =       bias_w_b_estim(1,1);        % estimate of bias of p-dir of angular velocity w
    bias_wq     =       bias_w_b_estim(2,1);        % estimate of bias of q-dir of angular velocity w
    bias_wr     =       bias_w_b_estim(3,1);        % estimate of bias of r-dir of angular velocity w
    % integration loop
    Nstep       = floor(Ts_EKF_meas/Ts_EKF_integr); % number of integration steps to performe in the t_meas time windows
    xt          = zeros(1,1);
    Pt          = zeros(1,1);
    for i = 1:1:Nstep
        % state extraction
            psi         =       xt1(1,1);           % roll angle (rad)
        
            cph         =       cos(phi);
            cth         =       cos(theta);
            cps         =       cos(psi);
            sph         =       sin(phi);
            sth         =       sin(theta);
            sps         =       sin(psi);
            tth         =       sth/cth;
        % integration
            Mf = [0,    sph/cth,    cph/cth,    0,  0,  0;];
            Z1 = [wp1-bias_wp; wq1-bias_wq; wr1-bias_wr; bias_wp; bias_wq; bias_wr;];
            f = Mf*Z1;
            xt = xt1 + Ts_EKF_integr*f;
        
            At1 = 0;
            Pt = Pt1 + Ts_EKF_integr*(At1*Pt1 + Pt1*At1' + Q);
        % house keeping
            xt1 = xt;
            Pt1 = Pt;
    end
  % MEASUREMENT STEP
    Ck = [eye(1)];
    Lk = Pt*Ck'/(Ck*Pt*Ck' + R);
    xk = xt + Lk*(Y_meas - Ck*xt);
    Pk = (eye(1) - Lk*Ck)*Pt;
else
    xk = xk1;
    Pk = Pk1;
end
end

== matlab function controller_3dof/Observer/Y_computation ==
  data: mf_b input; RP_estim input; Y_meas output
function Y_meas    = Y_computation(mf_b,RP_estim)
% description:
% - a_b             = measured linear acceleration in body-frame
% - w_b             = measured angular velocity in body-frame
% - mf_b            = measured magnetic field in body-frame
% - mf              = measured magnetic field in body-inertia
% - a_b_disturbe    = linear velocity measurement-noise
% - w_b_disturbe    = angular velocity measurement-noise
% - mf_b_disturbe   = magnetic field measurement-noise

% -------------------------------------------------------------------------------------------
% observation: the following computation works only if the angles
% phi,theta,psy are withing angles (-pi/2,+pi/2) (this is an open set, pi/2 is excluded)
% -------------------------------------------------------------------------------------------

ph_estim = RP_estim(1,1);
th_estim = RP_estim(2,1);

sph = sin(ph_estim);
cph = cos(ph_estim);

sth = sin(th_estim);
cth = cos(th_estim);

ps_meas_num   = mf_b(3)*sph - mf_b(2)*cph;
ps_meas_den = mf_b(1)*cth + mf_b(2)*sth*sph + mf_b(3)*sth*cph;
ps_meas = atan2(ps_meas_num, ps_meas_den);

if ps_meas < 0
    ps_meas = ps_meas + 2*pi;
end

Y_meas = ps_meas;
end

== matlab function controller_3dof/unlimited RPY/unlimited RPY ==
  data: RPY input; RPY output; RPY1 input; init output; init input
function [RPY,init] = unlimited_RPY(RPY,RPY1, init)
if init == 0
    init = 1;
    RPY1 = RPY;
end

for i =1:1:3
    while abs(RPY(i) - RPY1(i)) > pi/2
        RPY(i) = RPY(i) + sign(RPY1(i))*pi;
    end
end
end

== matlab function controller_3dof/Subsystem/MATLAB Function7 ==
  data: u input; y1 output; y2 output; y3 output
function [y1,y2,y3] = fcn(u)

y1 = u(1);
y2 = u(2);
y3 = u(3);

== matlab function controller_3dof/unlimited RPY2/unlimited RPY ==
  data: RPY input; RPY output; RPY1 input; init output; init input
function [RPY,init] = unlimited_RPY(RPY,RPY1, init)
if init == 0
    init = 1;
    RPY1 = RPY;
end

for i =1:1:3
    while abs(RPY(i) - RPY1(i)) > pi/2
        RPY(i) = RPY(i) + sign(RPY1(i))*pi;
    end
end
end

== matlab function controller_3dof/Subsystem/unlimited RPY1/unlimited RPY ==
  data: RPY input; RPY output; RPY1 input; init output; init input
function [RPY,init] = unlimited_RPY(RPY,RPY1, init)
if init == 0
    init = 1;
    RPY1 = RPY;
end

for i =1:1:3
    while abs(RPY(i) - RPY1(i)) > pi/2
        RPY(i) = RPY(i) + sign(RPY1(i))*pi;
    end
end
end

== matlab function controller_3dof/Subsystem/MATLAB Function1 ==
  data: u input; y1 output; y2 output; y3 output
function [y1,y2,y3] = fcn(u)

y1 = u(1);
y2 = u(2);
y3 = u(3);

== matlab function controller_3dof/MATLAB Function1 ==
  data: u input; y1 output; y2 output; y3 output
function [y1,y2,y3] = fcn(u)

y1 = u(1);
y2 = u(2);
y3 = u(3);

== matlab function controller_3dof/MATLAB Function3 ==
  data: u input; y1 output; y2 output; y3 output
function [y1,y2,y3] = fcn(u)

y1 = u(1);
y2 = u(2);
y3 = u(3);

== matlab function controller_3dof/MATLAB Function2 ==
  data: u_vect input; u1 output; u2 output; u3 output; u4 output
function [u1,u2,u3,u4] = fcn(u_vect)

u1 = u_vect(1);
u2 = u_vect(2);
u3 = u_vect(3);
u4 = u_vect(4);
end

== matlab function controller_3dof/IMU measurements & rotation/MATLAB Function ==
  data: u input; y output
function y = a_b_roation(u)
y = zeros(3,1);
y(1) = -u(1);
y(2) = +u(2);
y(3) = +u(3);
end

== matlab function controller_3dof/IMU measurements & rotation/MATLAB Function1 ==
  data: u input; y output
function y = w_b_roation(u)
y = zeros(3,1);
y(1) = +u(1);
y(2) = -u(2);
y(3) = -u(3);
end

== matlab function controller_3dof/Observer/MATLAB Function1 ==
  data: u input; y output
function y = fcn(u)

y = sqrt(u(1)^2 + u(2)^2 + u(3)^2);

== matlab function controller_3dof/allocation_logic ==
  data: tau input; u_max input; u output; tau_allocated output; u_min input; param parameter
function [u, tau_allocated] = allocation_logic(tau,u_max,u_min,param)
% Allocation Logic Block: computes the corresponding control command
% u = [u1,u2,u3,u4] given the torque command tau = [tau_phi, tau_theta, tau_phi]

% control command limits
%%u_min = 100;
% u_max = 1000;

l  = param(4,1);
k1 = param(5,1);
k2 = param(6,1);
k3 = param(7,1);
k4 = param(8,1);
b  = param(9,1);

u = zeros(4,1);
% [tau_ph; tau_th; tau_ps] = Mtau_u * [u1;u2;u3;u4]
Mtau_u = [0       0        l*k3    -l*k4;
         -l*k1    l*k2     0        0;
         -b      -b        b        b;];
% Minv = Mtau_u'*inv(Mtau_u*Mtau_u');
% up = Minv*tau;
% un = zeros(4,1);
% if min(up(:)) < u_min 
%     un = ones(4,1)*(u_min - min(up(:)));
% end
% u = up+un;
% for i = 1:1:4
%     if u(i,1) > u_max
%         u(i,1) = u_max;
%     end
% end
if tau(1) >= 0
    u(4) = u_min;
    u(3) = (tau(1) + l*k4*u(4))/(l*k3);
else
    u(3) = u_min;
    u(4) = (-tau(1) + l*k3*u(3))/(l*k4);
end
if tau(2) >= 0
    u(1) = u_min;
    u(2) = (tau(2) + l*k1*u(1))/(l*k2);
else
    u(2) = u_min;
    u(1) = (-tau(2) + l*k2*u(2))/(l*k1);
end
u = min(u_max,u);
tau_allocated = Mtau_u*u;

== matlab function controller_3dof/Observer/MATLAB Function2 ==
  data: u input; y output
function y = fcn(u)

y = sqrt(u(1)^2 + u(2)^2 + u(3)^2);

== matlab function controller_3dof/PX4/AQUISITION/MATLAB Function ==
  data: u input; y1 output; y2 output; y3 output; y4 output; y5 output; y6 output
function [y1,y2,y3,y4,y5,y6] = fcn(u)

y1 = u(1);
y2 = u(2);
y3 = u(3);
y4 = u(4);
y5 = u(5);
y6 = u(6);
